simulink model "prob8"  (R2020b)
settings: Solver=VariableStepAuto  StartTime=0.0  StopTime=10.0  RelTol=1e-3
settings Model: Creator=nadee  LastModifiedBy=nadee

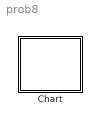
== system prob8 ==
  Chart : Stateflow chart  TreatAsAtomicUnit=on

== stateflow chart prob8/Chart ==
  state Stopped
    state Stopped_and_Waiting
      state Initializing
        entry: Motor = false; BrakesOff = false; Doors = false;
        DestinationReached = false; CommandConsidered = false;
      state FixingDestination
        LastDestination = WantedDestination;
      state SettingDown
        entry: Up = false;
      state SettingUp
        entry: Up = true
      state CommandAccepted
        CommandConsidered = true;
      (default) -> Initializing
      Initializing -> Initializing [order 2] : [~LiftCall && ~CommandConsidered]
      Initializing -> FixingDestination [order 1] : [LiftCall]
      FixingDestination -> SettingUp [order 1] : [CurrentPosition < LastDestination]
      FixingDestination -> SettingDown [order 2] : [CurrentPosition > LastDestination]
      SettingDown -> CommandAccepted
      SettingUp -> CommandAccepted
    state Stopped_at_Destination
      state StoppingLift
        entry: Motot = false; BrakesOff = false;
      state ErrorState
        entry: Doors = false;
      state OpeningDoors
        entry: DestinationReached = true; Doors = true
      (default) -> StoppingLift
      StoppingLift -> OpeningDoors [order 1] : [CurrenyPosition == LastDestination]
      StoppingLift -> ErrorState [order 2] : [CurrentPosition ~= LastDestination]
    (default) -> Stopped_and_Waiting
    Stopped_at_Destination -> Stopped_and_Waiting : [Doors]
    FixingDestination -> Stopped_at_Destination [order 3] : [CurrentPosition == LastDestination]
  state Moving
    state StartingMotor
  (default) -> Stopped
